simulink subsystem "CANOutputs"  (R2022b)
settings: Solver=VariableStepAuto  StartTime=0.0  StopTime=10.0  RelTol=1e-3
settings Model: Creator=serga  LastModifiedBy=serga

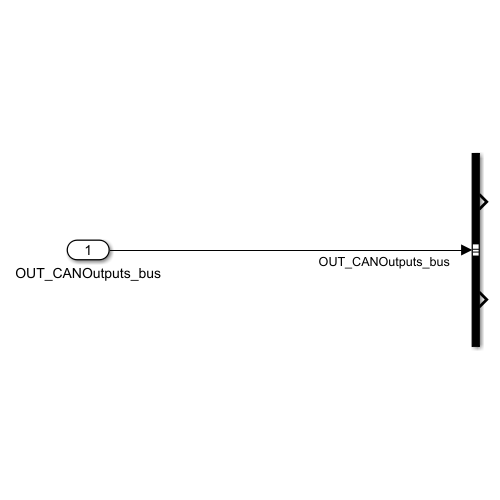
[thumbnail: Simulink's stored preview of the top-level diagram]
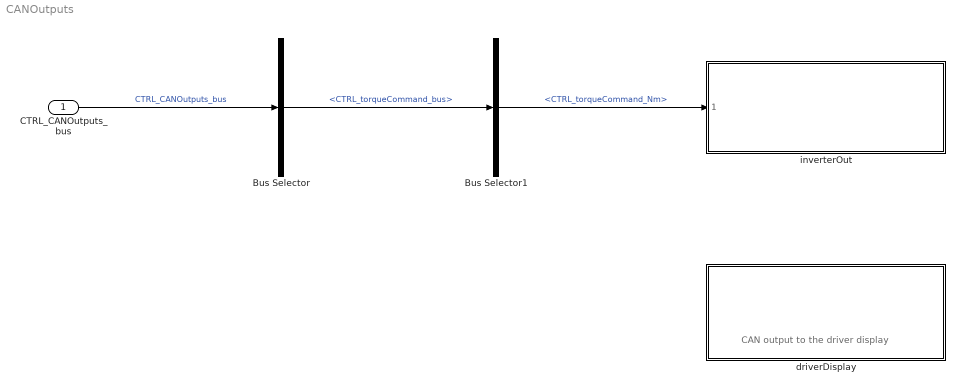
== system CANOutputs ==
  note: CAN output to the driver display
  CTRL_CANOutputs_bus : Inport
  Bus Selector : BusSelector  OutputSignals=CTRL_torqueCommand_bus
  Bus Selector1 : BusSelector  OutputSignals=CTRL_torqueCommand_Nm
  driverDisplay : Subsystem  ReferencedSubsystem=driverDisplay
  inverterOut : Subsystem  ReferencedSubsystem=inverterOut
  wires:
  CTRL_CANOutputs_bus/1 -> Bus Selector/1  "CTRL_CANOutputs_bus"
  Bus Selector/1 -> Bus Selector1/1  "<CTRL_torqueCommand_bus>"
  Bus Selector1/1 -> inverterOut/1  "<CTRL_torqueCommand_Nm>"
